simulink model "color_palette_v2"  (Simulink 7.6)
settings: Solver=FixedStepDiscrete  StartTime=0.0  StopTime=0  FixedStep=1/30  RelTol=1e-3
undefined symbols (not defined in the file or in its folder): jet, Rec, ref_colors, SDTV
libraries: vipconversions x1, vipsnks x1
settings Model: Creator=auvt  LastModifiedBy=auvt
settings RTWCC: TargetLang=C++

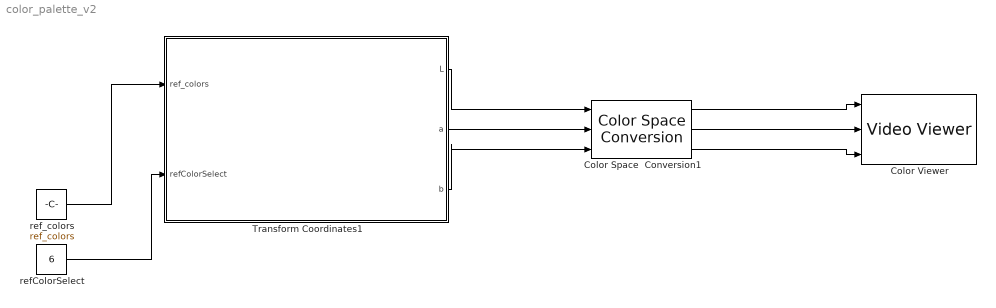
== system color_palette_v2 ==
  Color Space  Conversion1 : vipconversions/Color Space  Conversion  conversion=Obsolete  conversionActive=L*a*b* to sR'G'B'  wp_str=D50  rec=Rec. 601 (SDTV)  sys=1125/60/2:1  imagePorts=Separate color signals
  Color Viewer : vipsnks/Video Viewer  DialogControllerArgs=DataTag1  inputType=Obsolete7b  imagePorts=Separate color signals  useColorMap=off  colormapValue=jet(256)  specRange=off  minInputVal=0  maxInputVal=255  FigPos=[2049 844 410 300]  AxisZoom=on  trueSizedOnce=off  OpenAtMdlStart=on
  Transform Coordinates1 : Stateflow chart  TreatAsAtomicUnit=on  SystemSampleTime=[1/30 0]
  refColorSelect : Constant  Value=6  SampleTime=-1
  ref_colors : Constant  Value=ref_colors  SampleTime=-1
  wires:
  Transform Coordinates1/1(L) -> Color Space  Conversion1/1
  Transform Coordinates1/2(a) -> Color Space  Conversion1/2
  Transform Coordinates1/3(b) -> Color Space  Conversion1/3
  Color Space  Conversion1/1 -> Color Viewer/1
  Color Space  Conversion1/2 -> Color Viewer/2
  Color Space  Conversion1/3 -> Color Viewer/3
  refColorSelect/1 -> Transform Coordinates1/2(refColorSelect)
  ref_colors/1 -> Transform Coordinates1/1(ref_colors)

== matlab function Transform Coordinates1 ==
  data: L output double; a output double; b output double; ref_colors input double; refColorSelect input double
function [L, a, b] = makePalette(ref_colors, refColorSelect)


% Initialize
rows = 200;
cols = 200;

L = zeros(rows, cols);
a = zeros(rows, cols);
b = zeros(rows, cols);


% Display the color
for r = 1:rows
    for c = 1:cols
        
        L(r,c) = ref_colors(refColorSelect, 1);
        a(r,c) = ref_colors(refColorSelect, 2);
        b(r,c) = ref_colors(refColorSelect, 3);
        
    end
end


return
